simulink model "mdaqdemo_encoder"  (R2014a)
settings: Solver=FixedStepDiscrete  StartTime=0.0  StopTime=inf  FixedStep=0.01  RelTol=1e-3
libraries: microdaq_lib x5, simulink x2
settings Model: SimulationMode=external  CovSFcnEnable=on  Creator=skibool  LastModifiedBy=skibool
settings DataIOCC: SignalLoggingSaveFormat=ModelDataLogs
settings OptimizationCC: OptimizeModelRefInitCode=on  LifeSpan=1
settings DebuggingCC: UnderspecifiedInitializationDetection=Classic  MultiTaskDSMMsg=warning  MultiTaskCondExecSysMsg=none  FrameProcessingCompatibilityMsg=error
settings HardwareCC: ProdBitPerLong=40  ProdLargestAtomicInteger=Integer  ProdIntDivRoundTo=Zero  ProdEndianess=LittleEndian  ProdHWDeviceType=Texas Instruments->C6000
settings SFSimCC: SimParseCustomCode=off
settings RTWCC: SystemTargetFile=microdaq.tlc  TemplateMakefile=microdaq.tmf  PostCodeGenCommand=microdaq_postcodegen(buildInfo)  Description=MicroDAQ Real-Time Measurement System
settings CodeAppCC: IgnoreCustomStorageClasses=off
settings STFCustomTargetCC: CodeReplacementLibrary=C89/C90 (ANSI)  ConcurrentExecutionCompliant=off  GeneratePreprocessorConditionals=Use local settings  CombineOutputUpdateFcns=on  ERTCustomFileBanners=on  SupportContinuousTime=off  SupportNonInlinedSFcns=off  MATLABClassNameForMDSCustomization=Simulink.SoftwareTarget.ERTCustomization  GRTInterface=off  SystemTargetFile=microdaq.tlc
settings ERTTargetCC: CodeReplacementLibrary=C89/C90 (ANSI)  GenerateSampleERTMain=off  ExtMode=on  ExtModeStaticAlloc=on  ExtModeMexArgs=getpref('microdaq','TargetIP') 1 4344  InlinedParameterPlacement=Hierarchical  ERTCustomFileTemplate=microdaq_main.tlc

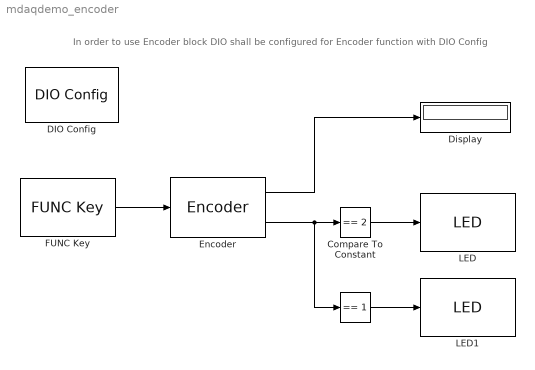
== system mdaqdemo_encoder ==
  note: In order to use Encoder block DIO shall be configured for Encoder function with DIO Config
  " " : simulink/Logic and Bit Operations/Compare To Constant  relop===  const=1  OutDataTypeStr=uint8
  Compare To Constant : simulink/Logic and Bit Operations/Compare To Constant  relop===  const=2  OutDataTypeStr=uint8
  DIO Config : microdaq_lib/Digital/DIO Config  enc1_func=Enable (DIO6 - Channel A, DIO8 - Channel B)  enc2_func=Disable  pwm1_func=Disable  pwm2_func=Disable  pwm3_func=Disable  dio1_dir=off  dio2_dir=off  dio3_dir=off  dio4_dir=off  dio5_dir=off  dio6_dir=off  dio7_dir=off  dio8_dir=off  dio9_dir=off  dio10_dir=off  dio11_dir=off  dio12_dir=off  dio13_dir=off  dio14_dir=off  dio15_dir=off  dio16_dir=off  dio17_dir=off  dio18_dir=off  dio19_dir=off  dio20_dir=off  dio21_dir=off  dio22_dir=off  dio23_dir=off  dio24_dir=off
  Display : Display
  Encoder : microdaq_lib/Motor Control/Encoder  pChannel=ENC1  SampleTime=0
  FUNC Key : microdaq_lib/Utilities/FUNC Key  pDIOFuncKey=F1  SampleTime=-1
  LED : microdaq_lib/Utilities/LED  SParameter1=D1
  LED1 : microdaq_lib/Utilities/LED  SParameter1=D2
  wires:
  Encoder/1 -> Display/1
  Encoder/2 -> " "/1, Compare To Constant/1
  Compare To Constant/1 -> LED/1
  " "/1 -> LED1/1
  FUNC Key/1 -> Encoder/1
